simulink model "fuzzytank"  (R2022b)
settings: Solver=VariableStepAuto  StartTime=0.0  StopTime=5.0  RelTol=1e-3
model workspace (MAT data in the model file):
  b = Simulink.Parameter
  b.Value = 0.5
  b.DataType = 'auto'
  b.Complexity = 'real'
  b.Dimensions = [1 1]
  h0 = Simulink.Parameter
  h0.Value = 2
  h0.DataType = 'auto'
  h0.Complexity = 'real'
  h0.Dimensions = [1 1]
  qe = Simulink.Parameter
  qe.Value = 1
  qe.DataType = 'auto'
  qe.Complexity = 'real'
  qe.Dimensions = [1 1]
libraries: fuzblock x1
settings Model: Creator=emmanuel  LastModifiedBy=emmanuel

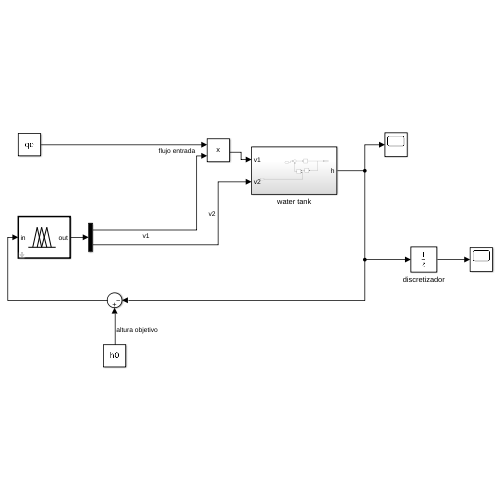
[thumbnail: Simulink's stored preview of the top-level diagram]
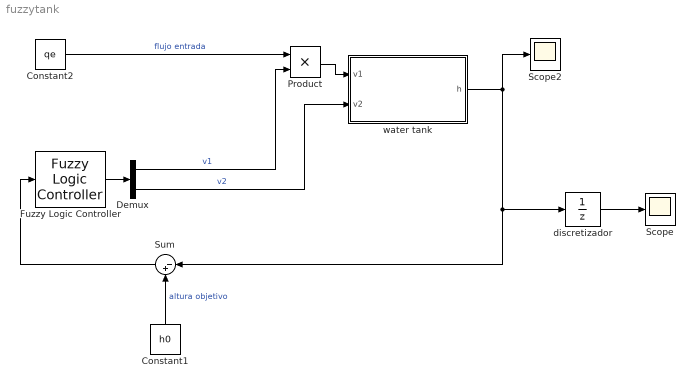
== system fuzzytank ==
  Constant1 : Constant  Value=h0
  Constant2 : Constant  Value=qe
  Demux : Demux  Outputs=2
  Fuzzy Logic Controller : fuzblock/Fuzzy Logic  Controller  FIS='error_tanque.fis'  OutputSampleNumber=101  DataType=double  FuzzifiedInputs=off  RuleFiringStrengths=off  RuleOutputs=off  AggregatedOutputs=off  SimulateUsing=Interpreted execution  OutOfRangeInputValueMessage=warning  NoRuleFiredMessage=warning  EmptyOutputFuzzySetMessage=warning
  Product : Product
  Scope : Scope
  Scope2 : Scope
  Sum : Sum  Inputs=|-+
  discretizador : UnitDelay  InitialCondition=4  SampleTime=0.1  HasFrameUpgradeWarning=on
  water tank : Subsystem
  wires:
  Constant2/1 -> Product/1  "flujo entrada"
  Sum/1 -> Fuzzy Logic Controller/1
  Constant1/1 -> Sum/2  "altura objetivo"
  Fuzzy Logic Controller/1 -> Demux/1
  Demux/1 -> Product/2  "v1"
  water tank/1(h) -> Scope2/1, discretizador/1, Sum/1
  Product/1 -> water tank/1(v1)
  Demux/2 -> water tank/2(v2)  "v2"
  discretizador/1 -> Scope/1

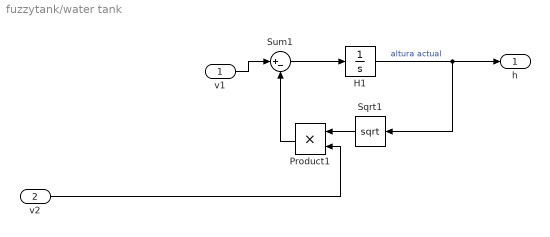
== system fuzzytank/water tank ==
  v1 : Inport
  v2 : Inport  Port=2
  H1 : Integrator  InitialCondition=4
  Product1 : Product
  Sqrt1 : Sqrt
  Sum1 : Sum  Inputs=|+-  SaturateOnIntegerOverflow=on
  h : Outport
  wires:
  Sqrt1/1 -> Product1/1
  Sum1/1 -> H1/1
  H1/1 -> Sqrt1/1, h/1  "altura actual"
  Product1/1 -> Sum1/2
  v1/1 -> Sum1/1
  v2/1 -> Product1/2
